simulink model "rst_auto_reg_complete_4a_2018b"  (R2018b)
settings: Solver=FixedStepAuto  StartTime=0.0  StopTime=200  RelTol=1e-3
values from neighbouring files (symbols this model uses):
  A = dend    [RST_2ordem_final.m]    (also in RST_4ordem_final.m)
  B = numd    [RST_2ordem_final.m]    (also in RST_4ordem_final.m)
  ep = 0.7    [RST_2ordem_final.m]    (also in RST_4ordem_final.m)
  initial_theta = [-0.31 -0.55 0.0021 0.12]    [RST_2ordem_final.m]    (also in RST_4ordem_final.m = [-1.0 0.38 0.07 0.23 0.03 0.12 0.06 0.005])
  Ta = 0.1    [RST_2ordem_final.m]    (also in RST_4ordem_final.m = 1)
  Tas = Ta    (= 0.1)    [RST_2ordem_final.m]    (also in RST_4ordem_final.m = 1)
  theta_switch_time = 10*Ta    (= 1)    [RST_2ordem_final.m]    (also in RST_4ordem_final.m = 10)
  Ts = 1    [RST_2ordem_final.m]    (also in RST_4ordem_final.m = 5)
  w0 = 1    [RST_2ordem_final.m]    (also in RST_4ordem_final.m = 0.1)
undefined symbols (not defined in the file or in its folder): R, S, T
libraries: dspinverses x6, simulink x2
(part 1 of 2)
settings Model: Creator=tarci  LastModifiedBy=root
settings DebuggingCC: LibraryContextMissingDiagnostic=none
settings SFSimCC: SimUseLocalCustomCode=off
settings RTWCC: RTWUseLocalCustomCode=off

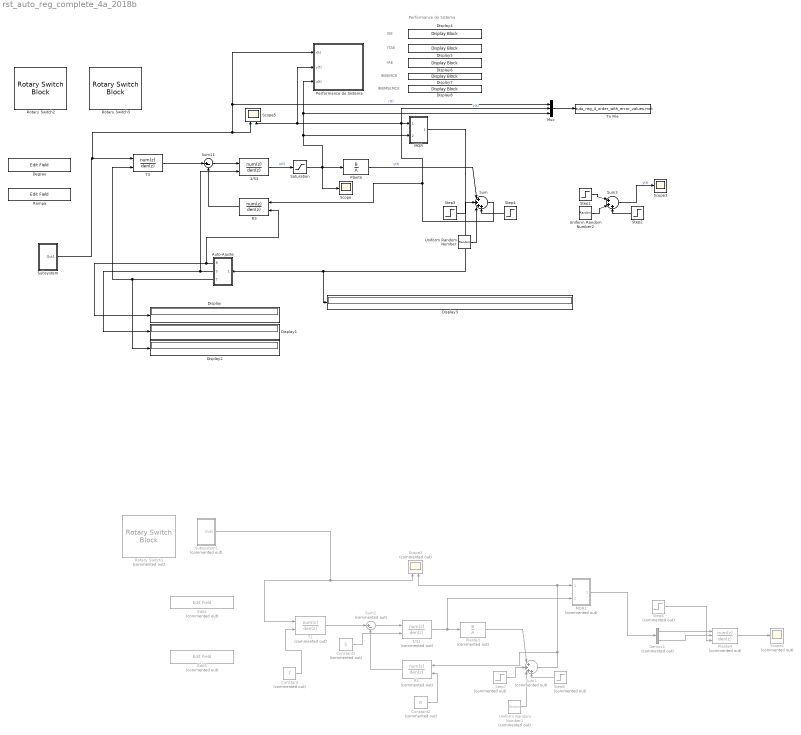
== system rst_auto_reg_complete_4a_2018b ==
  note: IRBEMCE
  note: IAE
  note: ITAE
  note: ISE
  note: Performance do Sistema
  note: IRBMSEMCE
  1/S1 : DiscreteFilter  Commented=on  Numerator=1  DenominatorSource=Input port  Denominator=1  SampleTime=Ta  a0EqualsOne=on
      settings: InputPortMap=u0,p3
  1/S3 : DiscreteFilter  Numerator=1  DenominatorSource=Input port  Denominator=1  SampleTime=Ta  a0EqualsOne=on
      settings: InputPortMap=u0,p3
  Auto-Ajuste : Subsystem
  Constant : Constant  Commented=on  Value=T
  Constant1 : Constant  Commented=on  Value=S
  Constant2 : Constant  Commented=on  Value=R
  Degrau : EditField  WebBlockId=1084  LabelPosition=Hide  Alignment=Center
  Demux1 : Demux  Commented=on  Outputs=2
  Display{,1..3} (4 alike) : Display
  Display4 : DisplayBlock  WebBlockId=2030  LabelPosition=Hide
  Display5 : DisplayBlock  WebBlockId=2031  LabelPosition=Hide
  Display6 : DisplayBlock  WebBlockId=2032  LabelPosition=Hide
  Display7 : DisplayBlock  WebBlockId=2033  LabelPosition=Hide
  Display8 : DisplayBlock  WebBlockId=2034  LabelPosition=Hide
  Edit2 : EditField  Commented=on  WebBlockId=1838  LabelPosition=Hide  Alignment=Center
  Edit3 : EditField  Commented=on  WebBlockId=1839  LabelPosition=Hide  Alignment=Center
  MQR : Subsystem
  MQR1 : Subsystem  Commented=on
  Mux : Mux  Inputs=3
  Performance do Sistema : Subsystem
  Planta : DiscreteFilter  Numerator=B  Denominator=A  SampleTime=Ta  a0EqualsOne=on
  Planta3 : DiscreteFilter  Commented=on  Numerator=B  Denominator=A  SampleTime=Ta  a0EqualsOne=on
  Planta4 : DiscreteFilter  Commented=on  NumeratorSource=Input port  Numerator=B  DenominatorSource=Input port  Denominator=A  SampleTime=Ta  a0EqualsOne=on
      settings: InputPortMap=u0,p1,p3
  R1 : DiscreteFilter  Commented=on  NumeratorSource=Input port  Numerator=[-620.2 131.3]  Denominator=1  SampleTime=Ta
      settings: InputPortMap=u0,p1
  R3 : DiscreteFilter  NumeratorSource=Input port  Numerator=[-620.2 131.3]  Denominator=1  SampleTime=Ta
      settings: InputPortMap=u0,p1
  Rampa : EditField  WebBlockId=1415  LabelPosition=Hide  Alignment=Center
  Rotary Switch1 : RotarySwitchBlock  Commented=on  WebBlockId=1942
      settings: Values={{'Degrau', 'Rampa', 'Senoide'}, [1 2 3]}
  Rotary Switch2 : RotarySwitchBlock  WebBlockId=1006
      settings: Values={{'Degrau', 'Rampa', 'Senoide'}, [1 2 3]}
  Rotary Switch3 : RotarySwitchBlock  WebBlockId=1934
      settings: Values={{'Degrau', 'Rampa', 'Senoide'}, [1 2 3]}
  Saturation : Saturate  UpperLimit=41  LowerLimit=0
  Scope : Scope
  Scope1 : Scope  Commented=on
  Scope2 : Scope  Commented=on  NumInputPorts=2
  Scope3 : Scope
  Scope5 : Scope  NumInputPorts=2
  Step1 : Step  Time=150  SampleTime=0
  Step2 : Step  Time=151  After=-1  SampleTime=0
  Step3 : Step  Time=150  SampleTime=0
  Step4 : Step  Time=151  After=-1  SampleTime=0
  Step6 : Step  Commented=on  SampleTime=0
  Step7 : Step  Commented=on  Time=40  SampleTime=0
  Step8 : Step  Commented=on  Time=41  After=-1  SampleTime=0
  Subsystem : Subsystem
  Subsystem1 : Subsystem  Commented=on
  Sum : Sum  Inputs=|++++
  Sum1 : Sum  Commented=on  Inputs=|++++
  Sum11 : Sum  Inputs=|+-
  Sum2 : Sum  Commented=on  Inputs=|+-
  Sum3 : Sum  Inputs=|+++
  T1 : DiscreteFilter  Commented=on  NumeratorSource=Input port  Numerator=13.39  Denominator=1  SampleTime=Ta
      settings: InputPortMap=u0,p1
  T3 : DiscreteFilter  NumeratorSource=Input port  Numerator=13.39  Denominator=1  SampleTime=Ta
      settings: InputPortMap=u0,p1
  To File : ToFile  Filename=auto_reg_4_order_with_error_values.mat
  Uniform Random Number : UniformRandomNumber  Minimum=-0.1  Maximum=0.1  Seed=10  SampleTime=0
  Uniform Random Number1 : UniformRandomNumber  Commented=on  Minimum=-0.1  Maximum=0.1  SampleTime=0
  Uniform Random Number2 : UniformRandomNumber  Minimum=-0.1  Maximum=0.1  Seed=10  SampleTime=0
  wires:
  Sum11/1 -> 1/S3/1
  R3/1 -> Sum11/2
  T3/1 -> Sum11/1
  Auto-Ajuste/1(R) -> Display/1, R3/2
  Auto-Ajuste/2(S) -> Display1/1, 1/S3/2
  Auto-Ajuste/3(T) -> Display2/1, T3/2
  MQR/1("Theta(t) ") -> Display3/1, Auto-Ajuste/1(Theta)
  Step3/1 -> Sum/2
  Step4/1 -> Sum/4
  Uniform Random Number/1 -> Sum/3
  Step8/1 -> Sum1/4
  Step7/1 -> Sum1/2
  1/S1/1 -> MQR1/2("u(t) "), Planta3/1
  Uniform Random Number1/1 -> Sum1/3
  Step6/1 -> Planta4/1
  Planta4/1 -> Scope1/1
  Demux1/2 -> Planta4/2
  Sum1/1 -> R1/1, Scope2/2, MQR1/1(y(t))
  R1/1 -> Sum2/2
  Subsystem1/1(Out1) -> T1/1, Scope2/1
  T1/1 -> Sum2/1
  Demux1/1 -> Planta4/3
  Sum2/1 -> 1/S1/1
  MQR1/1("Theta(t) ") -> Demux1/1
  Planta3/1 -> Sum1/1
  Constant/1 -> T1/2
  Constant1/1 -> 1/S1/2
  Constant2/1 -> R1/2
  Subsystem/1(Out1) -> Performance do Sistema/1(r(t)), Mux/1, Scope5/1, T3/1  "r(t)"
  1/S3/1 -> Saturation/1  "u(t)"
  Mux/1 -> To File/1
  Saturation/1 -> MQR/2("u(t) "), Mux/3, Performance do Sistema/3(u(t)), Planta/1, Scope/1
  Planta/1 -> Sum/1  "y(t)"
  Sum/1 -> R3/1, Scope5/2, Performance do Sistema/2(y(t)), Mux/2, MQR/1(y(t))  "y(t)"
  Step1/1 -> Sum3/1
  Uniform Random Number2/1 -> Sum3/2
  Step2/1 -> Sum3/3
  Sum3/1 -> Scope3/1  "y(t)"

== system rst_auto_reg_complete_4a_2018b/Auto-Ajuste ==
  Theta : Inport
  Damping3 : Constant  Value=ep
  Display : Display
  Display1 : Display
  Display2 : Display
  Frequência : Constant  Value=w0
  MC : Constant
  Multiport Switch : MultiPortSwitch
  Multiport Switch1 : MultiPortSwitch
  Multiport Switch2 : MultiPortSwitch
  RST Degrau : Subsystem
  RST Rampa : Subsystem
  RST Senoide : Subsystem
  Sample Time 2 : Constant  Value=Tas
  Sample Time3 : Constant  Value=Ta
  Ts3 : Constant  Value=Ts
  R : Outport
  S : Outport  Port=2
  T : Outport  Port=3
  wires:
  RST Senoide/4(L) -> Display2/1
  RST Degrau/4(L) -> Display1/1
  RST Rampa/2(S) -> Multiport Switch1/3
  RST Senoide/3(T) -> Multiport Switch2/4
  RST Rampa/4(L) -> Display/1
  Multiport Switch2/1 -> T/1
  Multiport Switch1/1 -> S/1
  Multiport Switch/1 -> R/1
  RST Senoide/1(R) -> Multiport Switch/4
  Ts3/1 -> RST Degrau/2(Ts), RST Rampa/2(Ts), RST Senoide/2(Ts)
  RST Degrau/2(S) -> Multiport Switch1/2
  RST Senoide/2(S) -> Multiport Switch1/4
  RST Rampa/1(R) -> Multiport Switch/3
  Frequência/1 -> RST Senoide/5(w0)
  Sample Time 2/1 -> RST Senoide/6(Tas)
  Sample Time3/1 -> RST Degrau/1(Sample Time), RST Rampa/1(Sample Time), RST Senoide/1(Sample Time)
  RST Rampa/3(T) -> Multiport Switch2/3
  Theta/1 -> RST Degrau/4(Theta), RST Rampa/4(Theta), RST Senoide/4(Theta)
  RST Degrau/3(T) -> Multiport Switch2/2
  Damping3/1 -> RST Degrau/3(Damping), RST Rampa/3(Damping), RST Senoide/3(Damping)
  RST Degrau/1(R) -> Multiport Switch/2
  MC/1 -> Multiport Switch/1, Multiport Switch1/1, Multiport Switch2/1

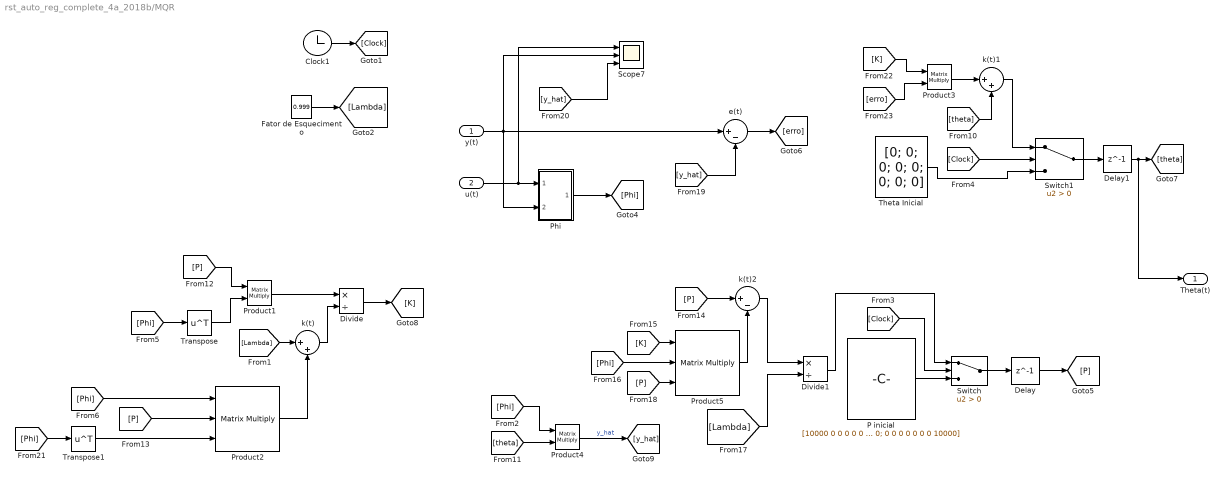
== system rst_auto_reg_complete_4a_2018b/MQR ==
  y(t) : Inport
  "u(t) " : Inport  Port=2
  Clock1 : Clock
  Delay : Delay  DelayLength=1  InitialCondition=0
  Delay1 : Delay  DelayLength=1  InitialCondition=0
  Divide : Product  Inputs=*/
  Divide1 : Product  Inputs=*/
  "Fator de Esquecimento " : Constant  Value=0.999
  P inicial : Constant  Value=[10000 0 0 0 0 0 0 0; 0 10000 0 0 0 0 0 0; 0 0 10000 0 0 0 0 0; 0 0 0 10000 0 0 0 0; 0 0 0 0 10000 0 0 0; 0 0 0 0 0 10000 0 0; 0 0 0 0 0 0 10000 0; 0 0 0 0 0 0 0 10000]
  Phi : Subsystem
  Product1 : Product  Multiplication=Matrix(*)
  Product2 : Product  Inputs=3  Multiplication=Matrix(*)
  Product3 : Product  Multiplication=Matrix(*)
  Product4 : Product  Multiplication=Matrix(*)
  Product5 : Product  Inputs=3  Multiplication=Matrix(*)
  Scope7 : Scope  NumInputPorts=3
  Switch : Switch  Criteria=u2 > Threshold
  Switch1 : Switch  Criteria=u2 > Threshold
  "Theta Inicial " : Constant  Value=[0; 0; 0; 0; 0; 0; 0; 0]
  Transpose : Math  Operator=transpose  SaturateOnIntegerOverflow=on
  Transpose1 : Math  Operator=transpose  SaturateOnIntegerOverflow=on
  e(t) : Sum  Inputs=|+-
  k(t) : Sum  Inputs=|++
  k(t)1 : Sum  Inputs=|++
  k(t)2 : Sum  Inputs=|+-
  "Theta(t) " : Outport
  wires:
  Product4/1 -> [y_hat]  "y_hat"
  [Phi] -> Product5/2
  Divide/1 -> [K]
  [Phi] -> Product2/1
  [P] -> Product1/1
  P inicial/1 -> Switch/3
  [K] -> Product5/1
  [y_hat] -> e(t)/2
  [erro] -> Product3/2
  Clock1/1 -> [Clock]
  Transpose/1 -> Product1/2
  [Lambda] -> k(t)/1
  [P] -> Product2/2
  [theta] -> k(t)1/2
  [P] -> k(t)2/1
  [theta] -> Product4/2
  [Clock] -> Switch/2
  [Phi] -> Transpose/1
  Divide1/1 -> Switch/1
  Transpose1/1 -> Product2/3
  "Theta Inicial "/1 -> Switch1/3
  "Fator de Esquecimento "/1 -> [Lambda]
  [P] -> Product5/3
  [Phi] -> Transpose1/1
  Delay/1 -> [P]
  Product3/1 -> k(t)1/1
  e(t)/1 -> [erro]
  Product1/1 -> Divide/1
  [Lambda] -> Divide1/2
  Switch/1 -> Delay/1
  "u(t) "/1 -> Phi/1(u(t)), Scope7/1
  Product5/1 -> k(t)2/2
  Delay1/1 -> [theta], "Theta(t) "/1
  k(t)2/1 -> Divide1/1
  y(t)/1 -> Phi/2(y(t)), Scope7/2, e(t)/1
  [Clock] -> Switch1/2
  Product2/1 -> k(t)/2
  [K] -> Product3/1
  Switch1/1 -> Delay1/1
  [y_hat] -> Scope7/3
  k(t)1/1 -> Switch1/1
  Phi/1(Phi) -> [Phi]
  [Phi] -> Product4/1
  k(t)/1 -> Divide/2

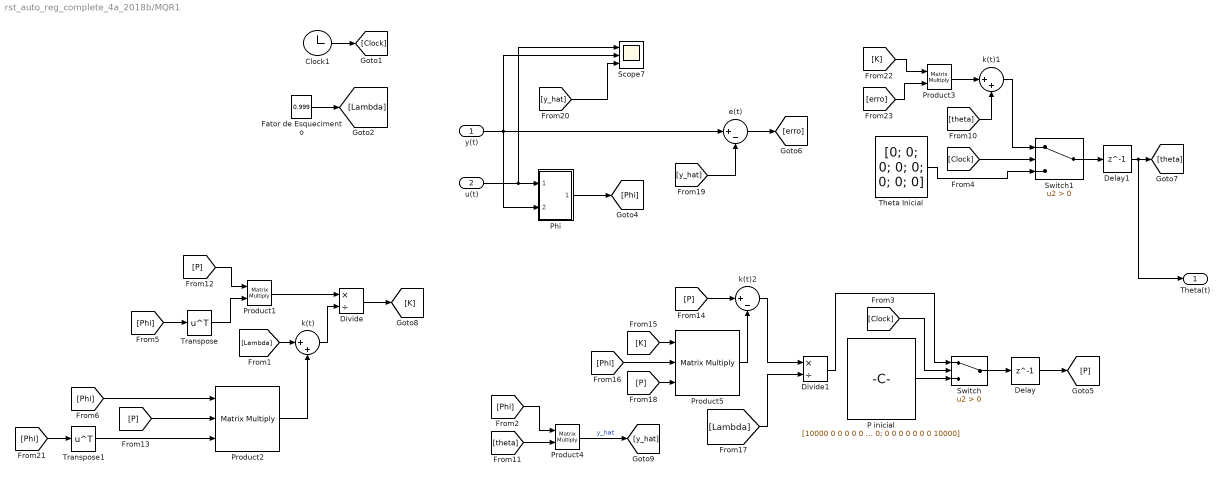
== system rst_auto_reg_complete_4a_2018b/MQR1 ==
  y(t) : Inport
  "u(t) " : Inport  Port=2
  Clock1 : Clock
  Delay : Delay  DelayLength=1  InitialCondition=0
  Delay1 : Delay  DelayLength=1  InitialCondition=0
  Divide : Product  Inputs=*/
  Divide1 : Product  Inputs=*/
  "Fator de Esquecimento " : Constant  Value=0.999
  P inicial : Constant  Value=[10000 0 0 0 0 0 0 0; 0 10000 0 0 0 0 0 0; 0 0 10000 0 0 0 0 0; 0 0 0 10000 0 0 0 0; 0 0 0 0 10000 0 0 0; 0 0 0 0 0 10000 0 0; 0 0 0 0 0 0 10000 0; 0 0 0 0 0 0 0 10000]
  Phi : Subsystem
  Product1 : Product  Multiplication=Matrix(*)
  Product2 : Product  Inputs=3  Multiplication=Matrix(*)
  Product3 : Product  Multiplication=Matrix(*)
  Product4 : Product  Multiplication=Matrix(*)
  Product5 : Product  Inputs=3  Multiplication=Matrix(*)
  Scope7 : Scope  NumInputPorts=3
  Switch : Switch  Criteria=u2 > Threshold
  Switch1 : Switch  Criteria=u2 > Threshold
  "Theta Inicial " : Constant  Value=[0; 0; 0; 0; 0; 0; 0; 0]
  Transpose : Math  Operator=transpose  SaturateOnIntegerOverflow=on
  Transpose1 : Math  Operator=transpose  SaturateOnIntegerOverflow=on
  e(t) : Sum  Inputs=|+-
  k(t) : Sum  Inputs=|++
  k(t)1 : Sum  Inputs=|++
  k(t)2 : Sum  Inputs=|+-
  "Theta(t) " : Outport
  wires:
  Product4/1 -> [y_hat]  "y_hat"
  [Phi] -> Product5/2
  Divide/1 -> [K]
  [Phi] -> Product2/1
  [P] -> Product1/1
  P inicial/1 -> Switch/3
  [K] -> Product5/1
  [y_hat] -> e(t)/2
  [erro] -> Product3/2
  Clock1/1 -> [Clock]
  Transpose/1 -> Product1/2
  [Lambda] -> k(t)/1
  [P] -> Product2/2
  [theta] -> k(t)1/2
  [P] -> k(t)2/1
  [theta] -> Product4/2
  [Clock] -> Switch/2
  [Phi] -> Transpose/1
  Divide1/1 -> Switch/1
  Transpose1/1 -> Product2/3
  "Theta Inicial "/1 -> Switch1/3
  "Fator de Esquecimento "/1 -> [Lambda]
  [P] -> Product5/3
  [Phi] -> Transpose1/1
  Delay/1 -> [P]
  Product3/1 -> k(t)1/1
  e(t)/1 -> [erro]
  Product1/1 -> Divide/1
  [Lambda] -> Divide1/2
  Switch/1 -> Delay/1
  "u(t) "/1 -> Phi/1(u(t)), Scope7/1
  Product5/1 -> k(t)2/2
  Delay1/1 -> [theta], "Theta(t) "/1
  k(t)2/1 -> Divide1/1
  y(t)/1 -> Phi/2(y(t)), Scope7/2, e(t)/1
  [Clock] -> Switch1/2
  Product2/1 -> k(t)/2
  [K] -> Product3/1
  Switch1/1 -> Delay1/1
  [y_hat] -> Scope7/3
  k(t)1/1 -> Switch1/1
  Phi/1(Phi) -> [Phi]
  [Phi] -> Product4/1
  k(t)/1 -> Divide/2

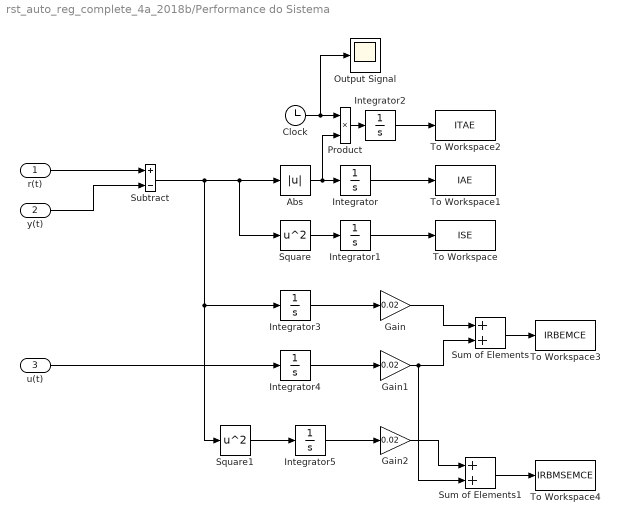
== system rst_auto_reg_complete_4a_2018b/Performance do Sistema ==
  r(t) : Inport
  y(t) : Inport  Port=2
  u(t) : Inport  Port=3
  Abs : Abs
  Clock : Clock
  Gain : Gain  Gain=0.02
  Gain1 : Gain  Gain=0.02
  Gain2 : Gain  Gain=0.02
  Integrator{,1..5} (6 alike) : Integrator
  Output Signal : Scope
  Product : Product
  Square : Math  Operator=square  SaturateOnIntegerOverflow=on
  Square1 : Math  Operator=square  SaturateOnIntegerOverflow=on
  Subtract : Sum  Inputs=+-
  Sum of Elements : Sum
  Sum of Elements1 : Sum
  To Workspace : ToWorkspace  VariableName=ISE  SaveFormat=Timeseries  SampleTime=-1
  To Workspace1 : ToWorkspace  VariableName=IAE  SaveFormat=Timeseries  SampleTime=-1
  To Workspace2 : ToWorkspace  VariableName=ITAE  SaveFormat=Timeseries  SampleTime=-1
  To Workspace3 : ToWorkspace  VariableName=IRBEMCE  SaveFormat=Timeseries  SampleTime=-1
  To Workspace4 : ToWorkspace  VariableName=IRBMSEMCE  SaveFormat=Timeseries  SampleTime=-1
  wires:
  y(t)/1 -> Subtract/2
  Abs/1 -> Product/2, Integrator/1
  Integrator/1 -> To Workspace1/1
  Integrator1/1 -> To Workspace/1
  Square/1 -> Integrator1/1
  Clock/1 -> Output Signal/1, Product/1
  Product/1 -> Integrator2/1
  Integrator2/1 -> To Workspace2/1
  r(t)/1 -> Subtract/1
  Subtract/1 -> Square1/1, Integrator3/1, Square/1, Abs/1
  Integrator3/1 -> Gain/1
  Integrator4/1 -> Gain1/1
  Gain/1 -> Sum of Elements/1
  Gain1/1 -> Sum of Elements1/2, Sum of Elements/2
  Square1/1 -> Integrator5/1
  Integrator5/1 -> Gain2/1
  Gain2/1 -> Sum of Elements1/1
  Sum of Elements/1 -> To Workspace3/1
  Sum of Elements1/1 -> To Workspace4/1
  u(t)/1 -> Integrator4/1

== system rst_auto_reg_complete_4a_2018b/Subsystem ==
  Constant3 : Constant
  Multiport Switch : MultiPortSwitch
  Ramp : simulink/Sources/Ramp  slope=1  start=1  InitialOutput=0
  Sine Wave : Sin  Frequency=w0  SampleTime=Tas
  Step1 : Step  Time=0  SampleTime=0
  Step2 : Step  Time=30  After=2  SampleTime=0
  Step3 : Step  Time=60  After=-3  SampleTime=0
  Step4 : Step  Time=90  After=4  SampleTime=0
  Step5 : Step  Time=120  After=-2  SampleTime=0
  Sum : Sum  Inputs=|+++++
  Out1 : Outport
  wires:
  Sine Wave/1 -> Multiport Switch/4
  Sum/1 -> Multiport Switch/2
  Constant3/1 -> Multiport Switch/1
  Ramp/1 -> Multiport Switch/3
  Multiport Switch/1 -> Out1/1
  Step2/1 -> Sum/2
  Step3/1 -> Sum/3
  Step1/1 -> Sum/1
  Step5/1 -> Sum/5
  Step4/1 -> Sum/4

== system rst_auto_reg_complete_4a_2018b/Subsystem1 ==
  C2 : Constant  Value=2
  Multiport Switch : MultiPortSwitch
  Ramp : simulink/Sources/Ramp  slope=1  start=1  InitialOutput=0
  Sine Wave : Sin  Frequency=w0  SampleTime=Tas
  Step1 : Step  Time=0  SampleTime=0
  Out1 : Outport
  wires:
  Multiport Switch/1 -> Out1/1
  Ramp/1 -> Multiport Switch/3
  C2/1 -> Multiport Switch/1
  Step1/1 -> Multiport Switch/2
  Sine Wave/1 -> Multiport Switch/4

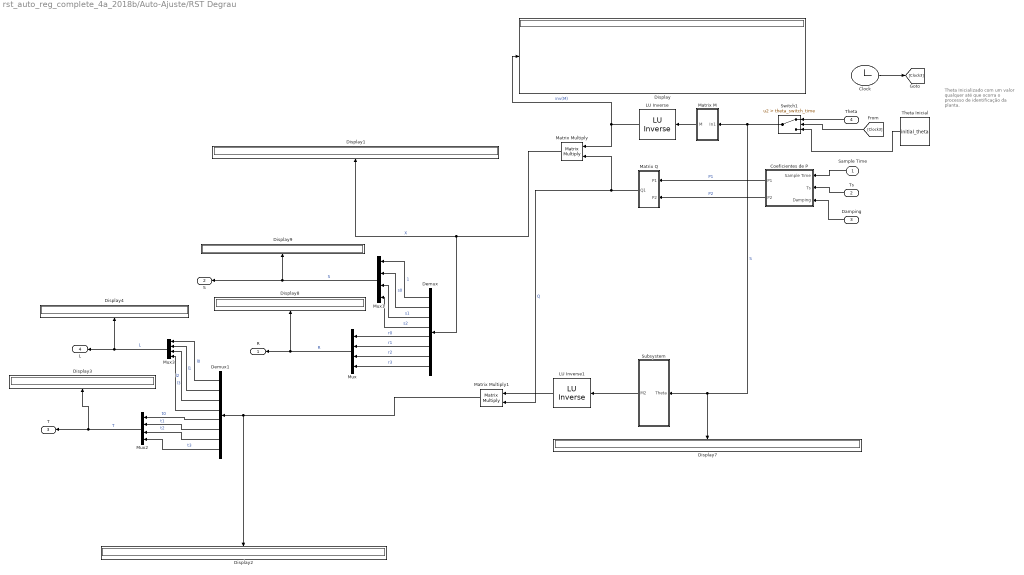
== system rst_auto_reg_complete_4a_2018b/Auto-Ajuste/RST Degrau ==
  note: Theta Inicializado com um
      | valor qualquer até que ocorra
      |  o processo de identificação
      | da planta.
  Sample Time : Inport
  Ts : Inport  Port=2
  Damping : Inport  Port=3
  Theta : Inport  Port=4
  " LU Inverse" : dspinverses/ LU Inverse
      settings: SourceProductName=DSP System Toolbox
  " LU Inverse1" : dspinverses/ LU Inverse
      settings: SourceProductName=DSP System Toolbox
  Clock : Clock
  Coeficientes de P : Subsystem
  Demux : Demux  Outputs=8
  Demux1 : Demux  Outputs=8
  Display{,1..4,7..9} (8 alike) : Display
  Matrix M : Subsystem
  Matrix Multiply : Product  Multiplication=Matrix(*)
  Matrix Multiply1 : Product  Multiplication=Matrix(*)
  Matrix Q : Subsystem
  Mux{,1..3} (4 alike) : Mux
  Subsystem : Subsystem
  Switch1 : Switch  Criteria=u2 > Threshold  Threshold=theta_switch_time
  Theta Inicial : Constant  Value=initial_theta
  R : Outport
  S : Outport  Port=2
  T : Outport  Port=3
  L : Outport  Port=4
  wires:
  Matrix Multiply1/1 -> Demux1/1, Display2/1
  Demux1/1 -> Mux3/1  "l0"
  Mux3/1 -> Display4/1, L/1  "L"
  Demux1/2 -> Mux3/2  "l1"
  Mux2/1 -> Display3/1, T/1  "T"
  Subsystem/1(M2) -> " LU Inverse1"/1
  Matrix Q/1(Q1) -> Matrix Multiply/2, Matrix Multiply1/2  "Q"
  " LU Inverse1"/1 -> Matrix Multiply1/1
  Demux/2 -> Mux1/2  "s0"
  Demux/1 -> Mux1/1  "1"
  Matrix M/1(M) -> " LU Inverse"/1
  Theta Inicial/1 -> Switch1/3
  [Clock3] -> Switch1/2
  Theta/1 -> Switch1/1
  Switch1/1 -> Subsystem/1(Theta), Display7/1, Matrix M/1(In1)  "S"
  Clock/1 -> [Clock3]
  Mux/1 -> Display8/1, R/1  "R"
  Coeficientes de P/1(P1) -> Matrix Q/1(P1)  "P1"
  Sample Time/1 -> Coeficientes de P/1(Sample Time)
  Damping/1 -> Coeficientes de P/3(Damping)
  Ts/1 -> Coeficientes de P/2(Ts)
  Coeficientes de P/2(P2) -> Matrix Q/2(P2)  "P2"
  Mux1/1 -> S/1, Display9/1  "S"
  " LU Inverse"/1 -> Display/1, Matrix Multiply/1  "inv(M)"
  Matrix Multiply/1 -> Display1/1, Demux/1  "X"
  Demux/3 -> Mux1/3  "s1"
  Demux/4 -> Mux1/4  "s2"
  Demux/5 -> Mux/1  "r0"
  Demux/6 -> Mux/2  "r1"
  Demux/7 -> Mux/3  "r2"
  Demux/8 -> Mux/4  "r3"
  Demux1/3 -> Mux3/3  "l2"
  Demux1/4 -> Mux3/4  "l3"
  Demux1/5 -> Mux2/1  "t0"
  Demux1/6 -> Mux2/2  "t1"
  Demux1/7 -> Mux2/3  "t2"
  Demux1/8 -> Mux2/4  "t3"

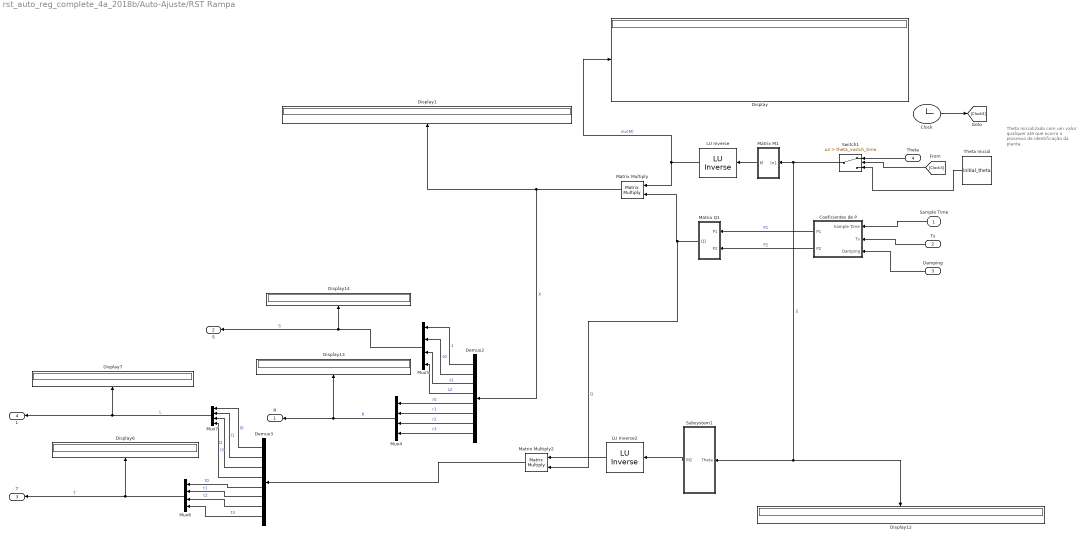
== system rst_auto_reg_complete_4a_2018b/Auto-Ajuste/RST Rampa ==
  note: Theta Inicializado com um
      | valor qualquer até que ocorra
      |  o processo de identificação
      | da planta.
  Sample Time : Inport
  Ts : Inport  Port=2
  Damping : Inport  Port=3
  Theta : Inport  Port=4
  " LU Inverse" : dspinverses/ LU Inverse
      settings: SourceProductName=DSP System Toolbox
  " LU Inverse2" : dspinverses/ LU Inverse
      settings: SourceProductName=DSP System Toolbox
  Clock : Clock
  Coeficientes de P : Subsystem
  Demux2 : Demux  Outputs=8
  Demux3 : Demux  Outputs=8
  Display{,1,6..7,12..14} (7 alike) : Display
  Matrix M1 : Subsystem
  Matrix Multiply : Product  Multiplication=Matrix(*)
  Matrix Multiply2 : Product  Multiplication=Matrix(*)
  Matrix Q1 : Subsystem
  Mux{4..7} (4 alike) : Mux
  Subsystem1 : Subsystem
  Switch1 : Switch  Criteria=u2 > Threshold  Threshold=theta_switch_time
  Theta Inicial : Constant  Value=initial_theta
  R : Outport
  S : Outport  Port=2
  T : Outport  Port=3
  L : Outport  Port=4
  wires:
  " LU Inverse"/1 -> Matrix Multiply/1, Display/1  "inv(M)"
  Coeficientes de P/2(P2) -> Matrix Q1/2(P2)  "P2"
  Ts/1 -> Coeficientes de P/2(Ts)
  Damping/1 -> Coeficientes de P/3(Damping)
  Sample Time/1 -> Coeficientes de P/1(Sample Time)
  Coeficientes de P/1(P1) -> Matrix Q1/1(P1)  "P1"
  Clock/1 -> [Clock3]
  Theta/1 -> Switch1/1
  [Clock3] -> Switch1/2
  Theta Inicial/1 -> Switch1/3
  Matrix M1/1(M) -> " LU Inverse"/1
  Demux3/3 -> Mux7/3  "l2"
  Demux2/8 -> Mux4/4  "r3"
  Demux2/5 -> Mux4/1  "r0"
  Demux2/4 -> Mux5/4  "s2"
  Demux3/2 -> Mux7/2  "l1"
  Demux2/3 -> Mux5/3  "s1"
  Demux3/8 -> Mux6/4  "t3"
  Demux3/5 -> Mux6/1  "t0"
  Mux4/1 -> Display13/1, R/1  "R"
  Switch1/1 -> Subsystem1/1(Theta), Display12/1, Matrix M1/1(In1)  "S"
  Demux2/2 -> Mux5/2  "s0"
  Mux5/1 -> Display14/1, S/1  "S"
  " LU Inverse2"/1 -> Matrix Multiply2/1
  Matrix Multiply/1 -> Demux2/1, Display1/1  "X"
  Demux3/7 -> Mux6/3  "t2"
  Demux2/1 -> Mux5/1  "1"
  Mux7/1 -> Display7/1, L/1  "L"
  Matrix Multiply2/1 -> Demux3/1
  Demux3/1 -> Mux7/1  "l0"
  Subsystem1/1(M2) -> " LU Inverse2"/1
  Matrix Q1/1(Q1) -> Matrix Multiply2/2, Matrix Multiply/2  "Q"
  Demux3/6 -> Mux6/2  "t1"
  Demux2/7 -> Mux4/3  "r2"
  Demux3/4 -> Mux7/4  "l3"
  Mux6/1 -> Display6/1, T/1  "T"
  Demux2/6 -> Mux4/2  "r1"

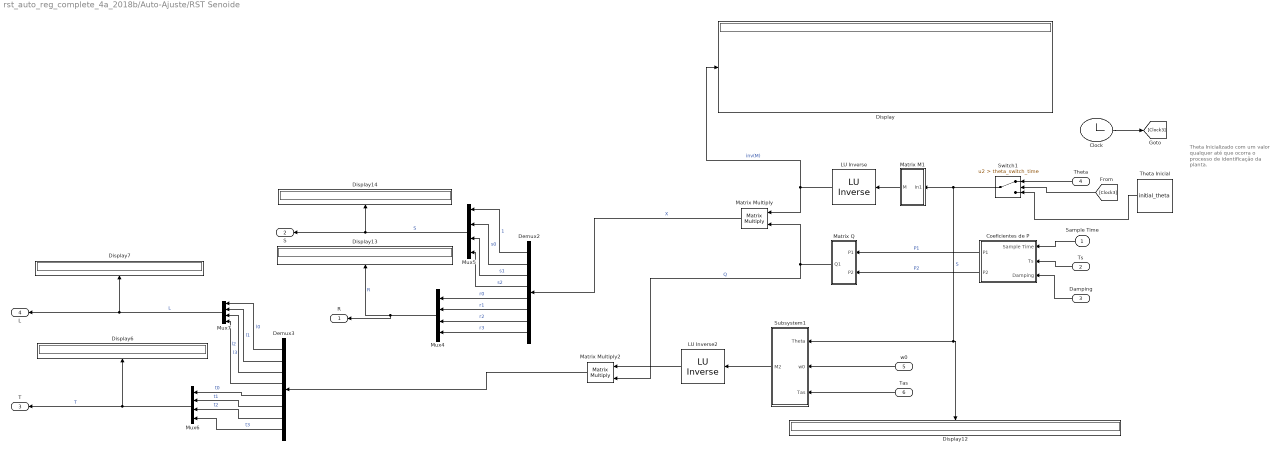
== system rst_auto_reg_complete_4a_2018b/Auto-Ajuste/RST Senoide ==
  note: Theta Inicializado com um
      | valor qualquer até que ocorra
      |  o processo de identificação
      | da planta.
  Sample Time : Inport
  Ts : Inport  Port=2
  Damping : Inport  Port=3
  Theta : Inport  Port=4
  w0 : Inport  Port=5
  Tas : Inport  Port=6
  " LU Inverse" : dspinverses/ LU Inverse
      settings: SourceProductName=DSP System Toolbox
  " LU Inverse2" : dspinverses/ LU Inverse
      settings: SourceProductName=DSP System Toolbox
  Clock : Clock
  Coeficientes de P : Subsystem
  Demux2 : Demux  Outputs=8
  Demux3 : Demux  Outputs=8
  Display{,6..7,12..14} (6 alike) : Display
  Matrix M1 : Subsystem
  Matrix Multiply : Product  Multiplication=Matrix(*)
  Matrix Multiply2 : Product  Multiplication=Matrix(*)
  Matrix Q : Subsystem
  Mux{4..7} (4 alike) : Mux
  Subsystem1 : Subsystem
  Switch1 : Switch  Criteria=u2 > Threshold  Threshold=theta_switch_time
  Theta Inicial : Constant  Value=initial_theta
  R : Outport
  S : Outport  Port=2
  T : Outport  Port=3
  L : Outport  Port=4
  wires:
  Tas/1 -> Subsystem1/3(Tas)
  w0/1 -> Subsystem1/2(w0)
  " LU Inverse"/1 -> Matrix Multiply/1, Display/1  "inv(M)"
  Coeficientes de P/2(P2) -> Matrix Q/2(P2)  "P2"
  Ts/1 -> Coeficientes de P/2(Ts)
  Damping/1 -> Coeficientes de P/3(Damping)
  Sample Time/1 -> Coeficientes de P/1(Sample Time)
  Coeficientes de P/1(P1) -> Matrix Q/1(P1)  "P1"
  Clock/1 -> [Clock3]
  Theta/1 -> Switch1/1
  [Clock3] -> Switch1/2
  Theta Inicial/1 -> Switch1/3
  Matrix M1/1(M) -> " LU Inverse"/1
  Demux3/3 -> Mux7/3  "l2"
  Demux2/8 -> Mux4/4  "r3"
  Demux2/5 -> Mux4/1  "r0"
  Demux2/4 -> Mux5/4  "s2"
  Demux3/2 -> Mux7/2  "l1"
  Demux2/3 -> Mux5/3  "s1"
  Demux3/8 -> Mux6/4  "t3"
  Demux3/5 -> Mux6/1  "t0"
  Mux4/1 -> Display13/1, R/1  "R"
  Switch1/1 -> Subsystem1/1(Theta), Display12/1, Matrix M1/1(In1)  "S"
  Demux2/2 -> Mux5/2  "s0"
  Mux5/1 -> Display14/1, S/1  "S"
  " LU Inverse2"/1 -> Matrix Multiply2/1
  Matrix Multiply/1 -> Demux2/1  "X"
  Demux3/7 -> Mux6/3  "t2"
  Demux2/1 -> Mux5/1  "1"
  Mux7/1 -> Display7/1, L/1  "L"
  Matrix Multiply2/1 -> Demux3/1
  Demux3/1 -> Mux7/1  "l0"
  Subsystem1/1(M2) -> " LU Inverse2"/1
  Matrix Q/1(Q1) -> Matrix Multiply/2, Matrix Multiply2/2  "Q"
  Demux3/6 -> Mux6/2  "t1"
  Demux2/7 -> Mux4/3  "r2"
  Demux3/4 -> Mux7/4  "l3"
  Mux6/1 -> Display6/1, T/1  "T"
  Demux2/6 -> Mux4/2  "r1"

== system rst_auto_reg_complete_4a_2018b/MQR/Phi ==
  u(t) : Inport
  y(t) : Inport  Port=2
  Constant : Constant  Value=-1
  Delay : Delay
  Delay1 : Delay  DelayLength=1
  Delay2 : Delay
  Delay3 : Delay  DelayLength=1
  Delay4 : Delay  DelayLength=3
  Delay5 : Delay  DelayLength=4
  Delay6 : Delay  DelayLength=3
  Delay7 : Delay  DelayLength=4
  Display : Display
  Product : Product
  Transpose1 : Math  Operator=transpose  SaturateOnIntegerOverflow=on
  Vector Concatenate : Concatenate  NumInputs=8
  Phi : Outport
  wires:
  Delay7/1 -> Vector Concatenate/8
  Delay6/1 -> Vector Concatenate/7
  Delay2/1 -> Vector Concatenate/6
  Delay3/1 -> Vector Concatenate/5
  Delay5/1 -> Vector Concatenate/4
  Delay4/1 -> Vector Concatenate/3
  Product/1 -> Delay1/1, Delay/1, Delay4/1, Delay5/1
  Constant/1 -> Product/2
  Transpose1/1 -> Phi/1
  Delay1/1 -> Vector Concatenate/1
  y(t)/1 -> Product/1
  Delay/1 -> Vector Concatenate/2
  Vector Concatenate/1 -> Display/1, Transpose1/1  "Phi"
  u(t)/1 -> Delay3/1, Delay2/1, Delay6/1, Delay7/1

== system rst_auto_reg_complete_4a_2018b/MQR1/Phi ==
  u(t) : Inport
  y(t) : Inport  Port=2
  Constant : Constant  Value=-1
  Delay : Delay
  Delay1 : Delay  DelayLength=1
  Delay2 : Delay
  Delay3 : Delay  DelayLength=1
  Delay4 : Delay  DelayLength=3
  Delay5 : Delay  DelayLength=4
  Delay6 : Delay  DelayLength=3
  Delay7 : Delay  DelayLength=4
  Display : Display
  Product : Product
  Transpose1 : Math  Operator=transpose  SaturateOnIntegerOverflow=on
  Vector Concatenate : Concatenate  NumInputs=8
  Phi : Outport
  wires:
  Delay7/1 -> Vector Concatenate/8
  Delay6/1 -> Vector Concatenate/7
  Delay2/1 -> Vector Concatenate/6
  Delay3/1 -> Vector Concatenate/5
  Delay5/1 -> Vector Concatenate/4
  Delay4/1 -> Vector Concatenate/3
  Product/1 -> Delay1/1, Delay/1, Delay4/1, Delay5/1
  Constant/1 -> Product/2
  Transpose1/1 -> Phi/1
  Delay1/1 -> Vector Concatenate/1
  y(t)/1 -> Product/1
  Delay/1 -> Vector Concatenate/2
  Vector Concatenate/1 -> Display/1, Transpose1/1  "Phi"
  u(t)/1 -> Delay3/1, Delay2/1, Delay6/1, Delay7/1

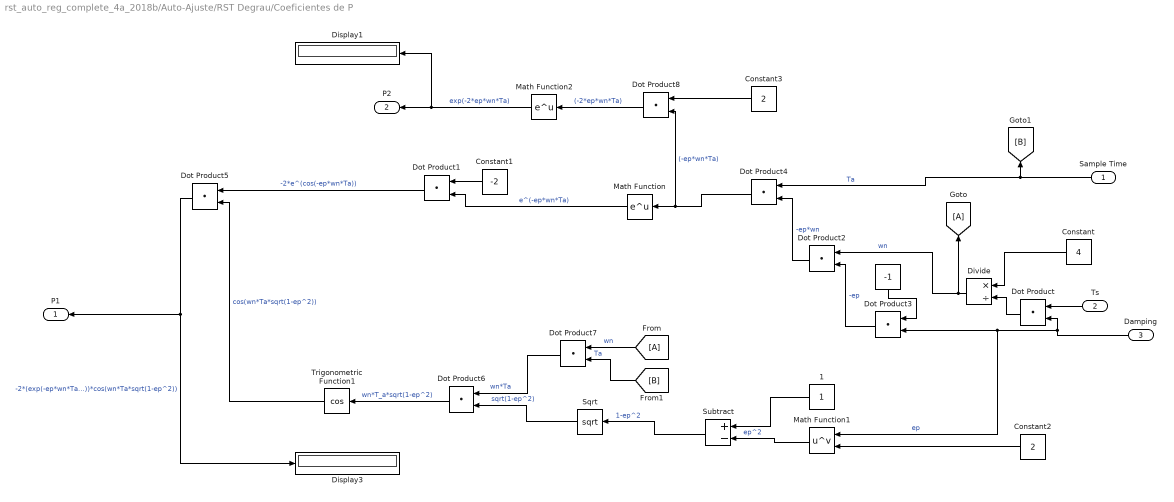
== system rst_auto_reg_complete_4a_2018b/Auto-Ajuste/RST Degrau/Coeficientes de P ==
  Sample Time : Inport
  Ts : Inport  Port=2
  Damping : Inport  Port=3
  " " : Constant  Value=-1
  1 : Constant
  Constant : Constant  Value=4
  Constant1 : Constant  Value=-2
  Constant2 : Constant  Value=2
  Constant3 : Constant  Value=2
  Display1 : Display
  Display3 : Display
  Divide : Product  Inputs=*/
  Dot Product{,1..8} (9 alike) : DotProduct  InputSameDT=on  OutDataTypeStr=Inherit: Inherit via internal rule
  Math Function : Math  SaturateOnIntegerOverflow=on
  Math Function1 : Math  Operator=pow  SaturateOnIntegerOverflow=on
  Math Function2 : Math  SaturateOnIntegerOverflow=on
  Sqrt : Sqrt  SaturateOnIntegerOverflow=on
  Subtract : Sum  Inputs=+-
  Trigonometric Function1 : Trigonometry  Operator=cos
  P1 : Outport
  P2 : Outport  Port=2
  wires:
  Math Function2/1 -> P2/1, Display1/1  "exp(-2*ep*wn*Ta)"
  Dot Product8/1 -> Math Function2/1  "(-2*ep*wn*Ta)"
  Constant3/1 -> Dot Product8/1
  Subtract/1 -> Sqrt/1  "1-ep^2"
  Sqrt/1 -> Dot Product6/2  "sqrt(1-ep^2)"
  Dot Product4/1 -> Math Function/1, Dot Product8/2  "(-ep*wn*Ta)"
  Dot Product6/1 -> Trigonometric Function1/1  "wn*T_a*sqrt(1-ep^2)"
  [B] -> Dot Product7/2  "Ta"
  Dot Product2/1 -> Dot Product4/2  "-ep*wn"
  Constant1/1 -> Dot Product1/1
  1/1 -> Subtract/1
  Constant2/1 -> Math Function1/2
  Dot Product1/1 -> Dot Product5/1  "-2*e^(cos(-ep*wn*Ta))"
  Math Function1/1 -> Subtract/2  "ep^2"
  Sample Time/1 -> [B], Dot Product4/1  "Ta"
  Dot Product7/1 -> Dot Product6/1  "wn*Ta"
  Constant/1 -> Divide/1
  Damping/1 -> Dot Product/2, Dot Product3/2, Math Function1/1  "ep"
  Dot Product3/1 -> Dot Product2/2  "-ep"
  Dot Product/1 -> Divide/2
  Ts/1 -> Dot Product/1
  Trigonometric Function1/1 -> Dot Product5/2  "cos(wn*Ta*sqrt(1-ep^2))"
  Dot Product5/1 -> Display3/1, P1/1  "-2*(exp(-ep*wn*Ta))*cos(wn*Ta*sqrt(1-ep^2))"
  " "/1 -> Dot Product3/1
  [A] -> Dot Product7/1  "wn"
  Divide/1 -> Dot Product2/1, [A]  "wn"
  Math Function/1 -> Dot Product1/2  "e^(-ep*wn*Ta)"

== system rst_auto_reg_complete_4a_2018b/Auto-Ajuste/RST Degrau/Matrix M ==
  In1 : Inport
  " 1" : Constant  Value=0
  2 : Constant
  Demux : Demux  Outputs=8
  Display1 : Display
  Matrix Concatenate{1..8} (8 alike) : Concatenate  NumInputs=8  Mode=Multidimensional array  ConcatenateDimension=2
  Matrix Concatenate{9..15} (7 alike) : Concatenate  Mode=Multidimensional array
  M : Outport
  wires:
  Matrix Concatenate12/1 -> Matrix Concatenate14/1
  Matrix Concatenate13/1 -> Matrix Concatenate14/2
  Matrix Concatenate6/1 -> Matrix Concatenate12/1
  2/1 -> Matrix Concatenate3/4, Matrix Concatenate2/3, Matrix Concatenate1/2, Matrix Concatenate6/1  "1"
  In1/1 -> Demux/1
  " 1"/1 -> Matrix Concatenate8/7, Matrix Concatenate8/6, Matrix Concatenate8/5, Matrix Concatenate8/3, Matrix Concatenate8/2, Matrix Concatenate8/1, Matrix Concatenate7/6, Matrix Concatenate7/5, Matrix Concatenate7/2, Matrix Concatenate7/1, Matrix Concatenate5/5, Matrix Concatenate5/1, Matrix Concatenate3/8, Matrix Concatenate2/8, Matrix Concatenate2/7, Matrix Concatenate2/4, Matrix Concatenate1/8, Matrix Concatenate1/7, Matrix Concatenate1/6, Matrix Concatenate1/4, Matrix Concatenate1/3, Matrix Concatenate6/8, Matrix Concatenate6/7, Matrix Concatenate6/6, Matrix Concatenate6/5, Matrix Concatenate6/4, Matrix Concatenate6/3, Matrix Concatenate6/2  "0"
  Demux/1 -> Matrix Concatenate4/4, Matrix Concatenate3/3, Matrix Concatenate2/2, Matrix Concatenate1/1  "a1"
  Demux/2 -> Matrix Concatenate5/4, Matrix Concatenate4/3, Matrix Concatenate3/2, Matrix Concatenate2/1  "a2"
  Demux/3 -> Matrix Concatenate7/4, Matrix Concatenate5/3, Matrix Concatenate4/2, Matrix Concatenate3/1  "a3"
  Demux/4 -> Matrix Concatenate8/4, Matrix Concatenate7/3, Matrix Concatenate5/2, Matrix Concatenate4/1  "a4"
  Demux/5 -> Matrix Concatenate4/8, Matrix Concatenate3/7, Matrix Concatenate2/6, Matrix Concatenate1/5  "b1"
  Demux/6 -> Matrix Concatenate5/8, Matrix Concatenate4/7, Matrix Concatenate3/6, Matrix Concatenate2/5  "b2"
  Demux/7 -> Matrix Concatenate7/8, Matrix Concatenate5/7, Matrix Concatenate4/6, Matrix Concatenate3/5  "b3"
  Demux/8 -> Matrix Concatenate8/8, Matrix Concatenate7/7, Matrix Concatenate5/6, Matrix Concatenate4/5  "b4"
  Matrix Concatenate1/1 -> Matrix Concatenate12/2
  Matrix Concatenate2/1 -> Matrix Concatenate13/1
  Matrix Concatenate3/1 -> Matrix Concatenate13/2
  Matrix Concatenate4/1 -> Matrix Concatenate9/1
  Matrix Concatenate5/1 -> Matrix Concatenate9/2
  Matrix Concatenate7/1 -> Matrix Concatenate10/1
  Matrix Concatenate8/1 -> Matrix Concatenate10/2
  Matrix Concatenate10/1 -> Matrix Concatenate11/2
  Matrix Concatenate9/1 -> Matrix Concatenate11/1
  Matrix Concatenate11/1 -> Matrix Concatenate15/2
  Matrix Concatenate14/1 -> Matrix Concatenate15/1
  Matrix Concatenate15/1 -> M/1, Display1/1

== system rst_auto_reg_complete_4a_2018b/Auto-Ajuste/RST Degrau/Matrix Q ==
  P1 : Inport
  P2 : Inport  Port=2
  Constant : Constant
  Constant1 : Constant  Value=0
  Display1 : Display
  Matrix Concatenate{1..7} (7 alike) : Concatenate  Mode=Multidimensional array
  Q1 : Outport
  wires:
  Constant1/1 -> Matrix Concatenate5/2, Matrix Concatenate5/1, Matrix Concatenate4/2, Matrix Concatenate4/1, Matrix Concatenate3/2
  Constant/1 -> Matrix Concatenate1/1
  P1/1 -> Matrix Concatenate1/2
  P2/1 -> Matrix Concatenate3/1
  Matrix Concatenate3/1 -> Matrix Concatenate2/2
  Matrix Concatenate1/1 -> Matrix Concatenate2/1
  Matrix Concatenate4/1 -> Matrix Concatenate6/1
  Matrix Concatenate5/1 -> Matrix Concatenate6/2
  Matrix Concatenate6/1 -> Matrix Concatenate7/2
  Matrix Concatenate2/1 -> Matrix Concatenate7/1
  Matrix Concatenate7/1 -> Q1/1, Display1/1

== system rst_auto_reg_complete_4a_2018b/Auto-Ajuste/RST Degrau/Subsystem ==
  Theta : Inport
  0 : Constant  Value=0
  Demux : Demux  Outputs=8
  Display1 : Display
  Display3 : Display
  Matrix Concatenate{1,9,16..21} (8 alike) : Concatenate  NumInputs=8  Mode=Multidimensional array  ConcatenateDimension=2
  Matrix Concatenate{3,7..8,10..11,15,22} (7 alike) : Concatenate  Mode=Multidimensional array
  Mux : Mux
  X1(1) : Constant
  X1(2) : Constant  Value=-1
  M2 : Outport
  wires:
  Matrix Concatenate1/1 -> Matrix Concatenate3/2
  Matrix Concatenate20/1 -> Matrix Concatenate10/1
  Matrix Concatenate21/1 -> Matrix Concatenate10/2
  Matrix Concatenate10/1 -> Matrix Concatenate11/2
  Matrix Concatenate11/1 -> Matrix Concatenate15/2
  Matrix Concatenate22/1 -> Matrix Concatenate11/1
  Matrix Concatenate18/1 -> Matrix Concatenate22/2
  Matrix Concatenate9/1 -> Matrix Concatenate7/1
  Matrix Concatenate17/1 -> Matrix Concatenate22/1
  Matrix Concatenate8/1 -> Matrix Concatenate15/1
  Matrix Concatenate16/1 -> Matrix Concatenate7/2
  Theta/1 -> Demux/1
  Matrix Concatenate3/1 -> Matrix Concatenate8/1
  Matrix Concatenate7/1 -> Matrix Concatenate8/2
  Matrix Concatenate19/1 -> Matrix Concatenate3/1
  X1(1)/1 -> Matrix Concatenate16/4, Matrix Concatenate9/3, Matrix Concatenate1/2, Matrix Concatenate19/1  "X1(1)"
  Demux/1 -> Mux/1  "a1"
  Demux/2 -> Mux/2  "a2"
  Demux/3 -> Mux/3  "a3"
  Demux/4 -> Mux/4  "a4"
  Mux/1 -> Display3/1
  0/1 -> Matrix Concatenate19/5, Matrix Concatenate1/6, Matrix Concatenate9/7, Matrix Concatenate16/8, Matrix Concatenate20/4, Matrix Concatenate21/7, Matrix Concatenate21/6, Matrix Concatenate21/5, Matrix Concatenate21/4, Matrix Concatenate21/3, Matrix Concatenate21/2, Matrix Concatenate21/1, Matrix Concatenate20/6, Matrix Concatenate20/5, Matrix Concatenate20/3, Matrix Concatenate20/2, Matrix Concatenate20/1, Matrix Concatenate18/5, Matrix Concatenate18/4, Matrix Concatenate18/3, Matrix Concatenate18/2, Matrix Concatenate18/1, Matrix Concatenate17/3, Matrix Concatenate17/2, Matrix Concatenate17/1, Matrix Concatenate16/2, Matrix Concatenate16/1, Matrix Concatenate9/8, Matrix Concatenate9/4, Matrix Concatenate9/1, Matrix Concatenate1/8, Matrix Concatenate1/7, Matrix Concatenate1/4, Matrix Concatenate1/3, Matrix Concatenate19/8, Matrix Concatenate19/7, Matrix Concatenate19/6, Matrix Concatenate19/4, Matrix Concatenate19/3, Matrix Concatenate19/2  "0"
  Matrix Concatenate15/1 -> M2/1, Display1/1
  X1(2)/1 -> Matrix Concatenate17/4, Matrix Concatenate16/3, Matrix Concatenate9/2, Matrix Concatenate1/1  "X1(2)"
  Demux/5 -> Matrix Concatenate17/8, Matrix Concatenate16/7, Matrix Concatenate9/6, Matrix Concatenate1/5  "b2"
  Demux/6 -> Matrix Concatenate18/8, Matrix Concatenate17/7, Matrix Concatenate16/6, Matrix Concatenate9/5  "b3"
  Demux/7 -> Matrix Concatenate20/8, Matrix Concatenate18/7, Matrix Concatenate17/6, Matrix Concatenate16/5  "b4"
  Demux/8 -> Matrix Concatenate21/8, Matrix Concatenate20/7, Matrix Concatenate18/6, Matrix Concatenate17/5  "b5"

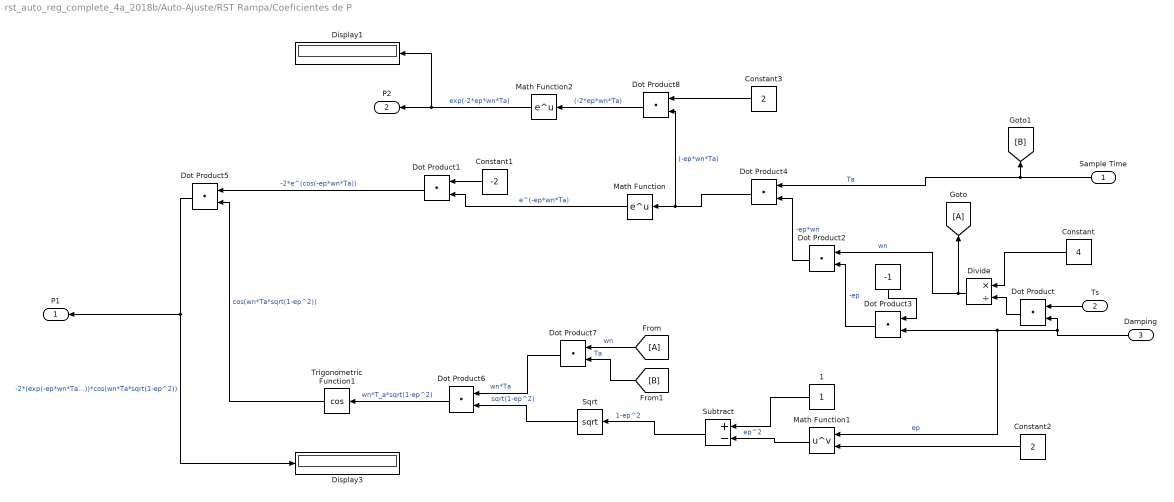
== system rst_auto_reg_complete_4a_2018b/Auto-Ajuste/RST Rampa/Coeficientes de P ==
  Sample Time : Inport
  Ts : Inport  Port=2
  Damping : Inport  Port=3
  " " : Constant  Value=-1
  1 : Constant
  Constant : Constant  Value=4
  Constant1 : Constant  Value=-2
  Constant2 : Constant  Value=2
  Constant3 : Constant  Value=2
  Display1 : Display
  Display3 : Display
  Divide : Product  Inputs=*/
  Dot Product{,1..8} (9 alike) : DotProduct  InputSameDT=on  OutDataTypeStr=Inherit: Inherit via internal rule
  Math Function : Math  SaturateOnIntegerOverflow=on
  Math Function1 : Math  Operator=pow  SaturateOnIntegerOverflow=on
  Math Function2 : Math  SaturateOnIntegerOverflow=on
  Sqrt : Sqrt  SaturateOnIntegerOverflow=on
  Subtract : Sum  Inputs=+-
  Trigonometric Function1 : Trigonometry  Operator=cos
  P1 : Outport
  P2 : Outport  Port=2
  wires:
  Math Function/1 -> Dot Product1/2  "e^(-ep*wn*Ta)"
  Divide/1 -> [A], Dot Product2/1  "wn"
  [A] -> Dot Product7/1  "wn"
  " "/1 -> Dot Product3/1
  Dot Product5/1 -> P1/1, Display3/1  "-2*(exp(-ep*wn*Ta))*cos(wn*Ta*sqrt(1-ep^2))"
  Trigonometric Function1/1 -> Dot Product5/2  "cos(wn*Ta*sqrt(1-ep^2))"
  Ts/1 -> Dot Product/1
  Dot Product/1 -> Divide/2
  Dot Product3/1 -> Dot Product2/2  "-ep"
  Damping/1 -> Math Function1/1, Dot Product3/2, Dot Product/2  "ep"
  Constant/1 -> Divide/1
  Dot Product7/1 -> Dot Product6/1  "wn*Ta"
  Sample Time/1 -> Dot Product4/1, [B]  "Ta"
  Math Function1/1 -> Subtract/2  "ep^2"
  Dot Product1/1 -> Dot Product5/1  "-2*e^(cos(-ep*wn*Ta))"
  Constant2/1 -> Math Function1/2
  1/1 -> Subtract/1
  Constant1/1 -> Dot Product1/1
  Dot Product2/1 -> Dot Product4/2  "-ep*wn"
  [B] -> Dot Product7/2  "Ta"
  Dot Product6/1 -> Trigonometric Function1/1  "wn*T_a*sqrt(1-ep^2)"
  Dot Product4/1 -> Dot Product8/2, Math Function/1  "(-ep*wn*Ta)"
  Sqrt/1 -> Dot Product6/2  "sqrt(1-ep^2)"
  Subtract/1 -> Sqrt/1  "1-ep^2"
  Constant3/1 -> Dot Product8/1
  Dot Product8/1 -> Math Function2/1  "(-2*ep*wn*Ta)"
  Math Function2/1 -> Display1/1, P2/1  "exp(-2*ep*wn*Ta)"

== system rst_auto_reg_complete_4a_2018b/Auto-Ajuste/RST Rampa/Matrix M1 ==
  In1 : Inport
  " 1" : Constant  Value=0
  2 : Constant
  Demux : Demux  Outputs=8
  Display1 : Display
  Matrix Concatenate{1..8} (8 alike) : Concatenate  NumInputs=8  Mode=Multidimensional array  ConcatenateDimension=2
  Matrix Concatenate{9..15} (7 alike) : Concatenate  Mode=Multidimensional array
  M : Outport
  wires:
  Matrix Concatenate12/1 -> Matrix Concatenate14/1
  Matrix Concatenate13/1 -> Matrix Concatenate14/2
  Matrix Concatenate6/1 -> Matrix Concatenate12/1
  2/1 -> Matrix Concatenate3/4, Matrix Concatenate2/3, Matrix Concatenate1/2, Matrix Concatenate6/1  "1"
  In1/1 -> Demux/1
  " 1"/1 -> Matrix Concatenate8/7, Matrix Concatenate8/6, Matrix Concatenate8/5, Matrix Concatenate8/3, Matrix Concatenate8/2, Matrix Concatenate8/1, Matrix Concatenate7/6, Matrix Concatenate7/5, Matrix Concatenate7/2, Matrix Concatenate7/1, Matrix Concatenate5/5, Matrix Concatenate5/1, Matrix Concatenate3/8, Matrix Concatenate2/8, Matrix Concatenate2/7, Matrix Concatenate2/4, Matrix Concatenate1/8, Matrix Concatenate1/7, Matrix Concatenate1/6, Matrix Concatenate1/4, Matrix Concatenate1/3, Matrix Concatenate6/8, Matrix Concatenate6/7, Matrix Concatenate6/6, Matrix Concatenate6/5, Matrix Concatenate6/4, Matrix Concatenate6/3, Matrix Concatenate6/2  "0"
  Demux/1 -> Matrix Concatenate4/4, Matrix Concatenate3/3, Matrix Concatenate2/2, Matrix Concatenate1/1  "a1"
  Demux/2 -> Matrix Concatenate5/4, Matrix Concatenate4/3, Matrix Concatenate3/2, Matrix Concatenate2/1  "a2"
  Demux/3 -> Matrix Concatenate7/4, Matrix Concatenate5/3, Matrix Concatenate4/2, Matrix Concatenate3/1  "a3"
  Demux/4 -> Matrix Concatenate8/4, Matrix Concatenate7/3, Matrix Concatenate5/2, Matrix Concatenate4/1  "a4"
  Demux/5 -> Matrix Concatenate4/8, Matrix Concatenate3/7, Matrix Concatenate2/6, Matrix Concatenate1/5  "b1"
  Demux/6 -> Matrix Concatenate5/8, Matrix Concatenate4/7, Matrix Concatenate3/6, Matrix Concatenate2/5  "b2"
  Demux/7 -> Matrix Concatenate7/8, Matrix Concatenate5/7, Matrix Concatenate4/6, Matrix Concatenate3/5  "b3"
  Demux/8 -> Matrix Concatenate8/8, Matrix Concatenate7/7, Matrix Concatenate5/6, Matrix Concatenate4/5  "b4"
  Matrix Concatenate1/1 -> Matrix Concatenate12/2
  Matrix Concatenate2/1 -> Matrix Concatenate13/1
  Matrix Concatenate3/1 -> Matrix Concatenate13/2
  Matrix Concatenate4/1 -> Matrix Concatenate9/1
  Matrix Concatenate5/1 -> Matrix Concatenate9/2
  Matrix Concatenate7/1 -> Matrix Concatenate10/1
  Matrix Concatenate8/1 -> Matrix Concatenate10/2
  Matrix Concatenate10/1 -> Matrix Concatenate11/2
  Matrix Concatenate9/1 -> Matrix Concatenate11/1
  Matrix Concatenate11/1 -> Matrix Concatenate15/2
  Matrix Concatenate14/1 -> Matrix Concatenate15/1
  Matrix Concatenate15/1 -> M/1, Display1/1

== system rst_auto_reg_complete_4a_2018b/Auto-Ajuste/RST Rampa/Matrix Q1 ==
  P1 : Inport
  P2 : Inport  Port=2
  Constant : Constant
  Constant1 : Constant  Value=0
  Display1 : Display
  Matrix Concatenate{1..7} (7 alike) : Concatenate  Mode=Multidimensional array
  Q1 : Outport
  wires:
  Constant1/1 -> Matrix Concatenate5/2, Matrix Concatenate5/1, Matrix Concatenate4/2, Matrix Concatenate4/1, Matrix Concatenate3/2
  Constant/1 -> Matrix Concatenate1/1
  P1/1 -> Matrix Concatenate1/2
  P2/1 -> Matrix Concatenate3/1
  Matrix Concatenate3/1 -> Matrix Concatenate2/2
  Matrix Concatenate1/1 -> Matrix Concatenate2/1
  Matrix Concatenate4/1 -> Matrix Concatenate6/1
  Matrix Concatenate5/1 -> Matrix Concatenate6/2
  Matrix Concatenate6/1 -> Matrix Concatenate7/2
  Matrix Concatenate2/1 -> Matrix Concatenate7/1
  Matrix Concatenate7/1 -> Q1/1, Display1/1

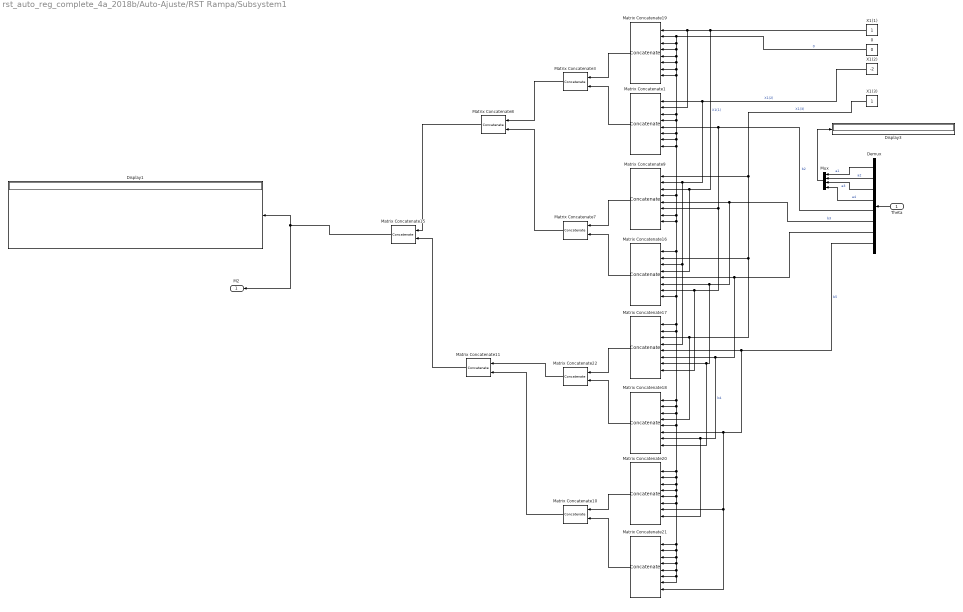
== system rst_auto_reg_complete_4a_2018b/Auto-Ajuste/RST Rampa/Subsystem1 ==
  Theta : Inport
  0 : Constant  Value=0
  Demux : Demux  Outputs=8
  Display1 : Display
  Display3 : Display
  Matrix Concatenate{1,9,16..21} (8 alike) : Concatenate  NumInputs=8  Mode=Multidimensional array  ConcatenateDimension=2
  Matrix Concatenate{3,7..8,10..11,15,22} (7 alike) : Concatenate  Mode=Multidimensional array
  Mux : Mux
  X1(1) : Constant
  X1(2) : Constant  Value=-2
  X1(3) : Constant
  M2 : Outport
  wires:
  Matrix Concatenate1/1 -> Matrix Concatenate3/2
  Matrix Concatenate20/1 -> Matrix Concatenate10/1
  Matrix Concatenate21/1 -> Matrix Concatenate10/2
  Matrix Concatenate10/1 -> Matrix Concatenate11/2
  Matrix Concatenate11/1 -> Matrix Concatenate15/2
  Matrix Concatenate22/1 -> Matrix Concatenate11/1
  Matrix Concatenate18/1 -> Matrix Concatenate22/2
  Matrix Concatenate9/1 -> Matrix Concatenate7/1
  Matrix Concatenate17/1 -> Matrix Concatenate22/1
  Matrix Concatenate8/1 -> Matrix Concatenate15/1
  Matrix Concatenate16/1 -> Matrix Concatenate7/2
  Theta/1 -> Demux/1
  Matrix Concatenate3/1 -> Matrix Concatenate8/1
  Matrix Concatenate7/1 -> Matrix Concatenate8/2
  Matrix Concatenate19/1 -> Matrix Concatenate3/1
  X1(1)/1 -> Matrix Concatenate16/4, Matrix Concatenate9/3, Matrix Concatenate1/2, Matrix Concatenate19/1  "X1(1)"
  Demux/1 -> Mux/1  "a1"
  Demux/2 -> Mux/2  "a2"
  Demux/3 -> Mux/3  "a3"
  Demux/4 -> Mux/4  "a4"
  Mux/1 -> Display3/1
  0/1 -> Matrix Concatenate19/5, Matrix Concatenate1/6, Matrix Concatenate9/7, Matrix Concatenate16/8, Matrix Concatenate20/4, Matrix Concatenate21/7, Matrix Concatenate21/6, Matrix Concatenate21/5, Matrix Concatenate21/4, Matrix Concatenate21/3, Matrix Concatenate21/2, Matrix Concatenate21/1, Matrix Concatenate20/6, Matrix Concatenate20/5, Matrix Concatenate20/3, Matrix Concatenate20/2, Matrix Concatenate20/1, Matrix Concatenate18/5, Matrix Concatenate18/3, Matrix Concatenate18/2, Matrix Concatenate18/1, Matrix Concatenate17/2, Matrix Concatenate17/1, Matrix Concatenate16/1, Matrix Concatenate9/8, Matrix Concatenate9/4, Matrix Concatenate1/8, Matrix Concatenate1/7, Matrix Concatenate1/4, Matrix Concatenate1/3, Matrix Concatenate19/8, Matrix Concatenate19/7, Matrix Concatenate19/6, Matrix Concatenate19/4, Matrix Concatenate19/3, Matrix Concatenate19/2  "0"
  Matrix Concatenate15/1 -> M2/1, Display1/1
  X1(2)/1 -> Matrix Concatenate17/4, Matrix Concatenate16/3, Matrix Concatenate9/2, Matrix Concatenate1/1  "X1(2)"
  Demux/5 -> Matrix Concatenate17/8, Matrix Concatenate16/7, Matrix Concatenate9/6, Matrix Concatenate1/5  "b2"
  Demux/6 -> Matrix Concatenate18/8, Matrix Concatenate17/7, Matrix Concatenate16/6, Matrix Concatenate9/5  "b3"
  Demux/7 -> Matrix Concatenate20/8, Matrix Concatenate18/7, Matrix Concatenate17/6, Matrix Concatenate16/5  "b4"
  Demux/8 -> Matrix Concatenate21/8, Matrix Concatenate20/7, Matrix Concatenate18/6, Matrix Concatenate17/5  "b5"
  X1(3)/1 -> Matrix Concatenate18/4, Matrix Concatenate17/3, Matrix Concatenate16/2, Matrix Concatenate9/1  "X1(3)"

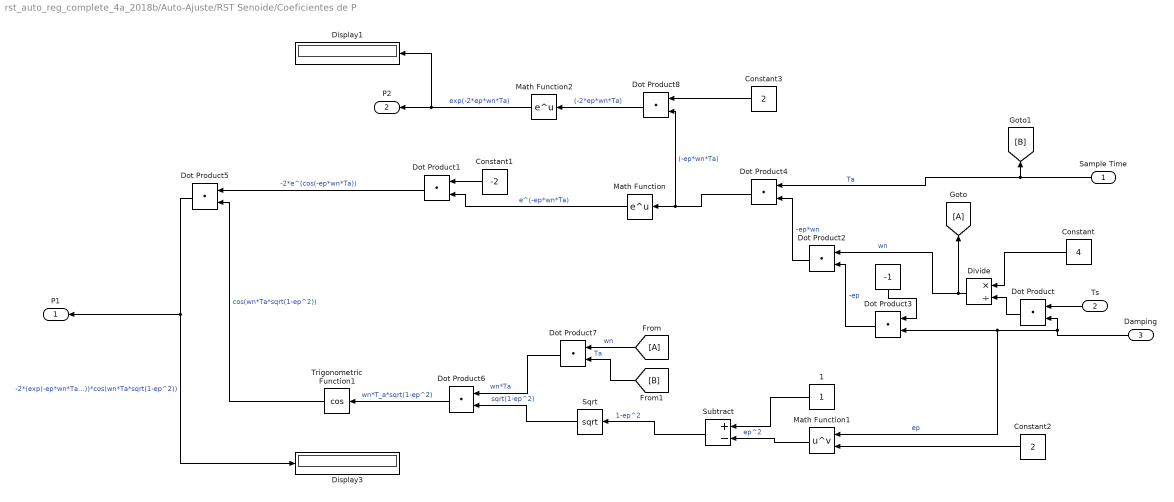
== system rst_auto_reg_complete_4a_2018b/Auto-Ajuste/RST Senoide/Coeficientes de P ==
  Sample Time : Inport
  Ts : Inport  Port=2
  Damping : Inport  Port=3
  " " : Constant  Value=-1
  1 : Constant
  Constant : Constant  Value=4
  Constant1 : Constant  Value=-2
  Constant2 : Constant  Value=2
  Constant3 : Constant  Value=2
  Display1 : Display
  Display3 : Display
  Divide : Product  Inputs=*/
  Dot Product{,1..8} (9 alike) : DotProduct  InputSameDT=on  OutDataTypeStr=Inherit: Inherit via internal rule
  Math Function : Math  SaturateOnIntegerOverflow=on
  Math Function1 : Math  Operator=pow  SaturateOnIntegerOverflow=on
  Math Function2 : Math  SaturateOnIntegerOverflow=on
  Sqrt : Sqrt  SaturateOnIntegerOverflow=on
  Subtract : Sum  Inputs=+-
  Trigonometric Function1 : Trigonometry  Operator=cos
  P1 : Outport
  P2 : Outport  Port=2
  wires:
  Math Function/1 -> Dot Product1/2  "e^(-ep*wn*Ta)"
  Divide/1 -> [A], Dot Product2/1  "wn"
  [A] -> Dot Product7/1  "wn"
  " "/1 -> Dot Product3/1
  Dot Product5/1 -> P1/1, Display3/1  "-2*(exp(-ep*wn*Ta))*cos(wn*Ta*sqrt(1-ep^2))"
  Trigonometric Function1/1 -> Dot Product5/2  "cos(wn*Ta*sqrt(1-ep^2))"
  Ts/1 -> Dot Product/1
  Dot Product/1 -> Divide/2
  Dot Product3/1 -> Dot Product2/2  "-ep"
  Damping/1 -> Math Function1/1, Dot Product3/2, Dot Product/2  "ep"
  Constant/1 -> Divide/1
  Dot Product7/1 -> Dot Product6/1  "wn*Ta"
  Sample Time/1 -> Dot Product4/1, [B]  "Ta"
  Math Function1/1 -> Subtract/2  "ep^2"
  Dot Product1/1 -> Dot Product5/1  "-2*e^(cos(-ep*wn*Ta))"
  Constant2/1 -> Math Function1/2
  1/1 -> Subtract/1
  Constant1/1 -> Dot Product1/1
  Dot Product2/1 -> Dot Product4/2  "-ep*wn"
  [B] -> Dot Product7/2  "Ta"
  Dot Product6/1 -> Trigonometric Function1/1  "wn*T_a*sqrt(1-ep^2)"
  Dot Product4/1 -> Dot Product8/2, Math Function/1  "(-ep*wn*Ta)"
  Sqrt/1 -> Dot Product6/2  "sqrt(1-ep^2)"
  Subtract/1 -> Sqrt/1  "1-ep^2"
  Constant3/1 -> Dot Product8/1
  Dot Product8/1 -> Math Function2/1  "(-2*ep*wn*Ta)"
  Math Function2/1 -> Display1/1, P2/1  "exp(-2*ep*wn*Ta)"

== system rst_auto_reg_complete_4a_2018b/Auto-Ajuste/RST Senoide/Matrix M1 ==
  In1 : Inport
  " 1" : Constant  Value=0
  2 : Constant
  Demux : Demux  Outputs=8
  Display1 : Display
  Matrix Concatenate{1..8} (8 alike) : Concatenate  NumInputs=8  Mode=Multidimensional array  ConcatenateDimension=2
  Matrix Concatenate{9..15} (7 alike) : Concatenate  Mode=Multidimensional array
  M : Outport
  wires:
  Matrix Concatenate12/1 -> Matrix Concatenate14/1
  Matrix Concatenate13/1 -> Matrix Concatenate14/2
  Matrix Concatenate6/1 -> Matrix Concatenate12/1
  2/1 -> Matrix Concatenate3/4, Matrix Concatenate2/3, Matrix Concatenate1/2, Matrix Concatenate6/1  "1"
  In1/1 -> Demux/1
  " 1"/1 -> Matrix Concatenate8/7, Matrix Concatenate8/6, Matrix Concatenate8/5, Matrix Concatenate8/3, Matrix Concatenate8/2, Matrix Concatenate8/1, Matrix Concatenate7/6, Matrix Concatenate7/5, Matrix Concatenate7/2, Matrix Concatenate7/1, Matrix Concatenate5/5, Matrix Concatenate5/1, Matrix Concatenate3/8, Matrix Concatenate2/8, Matrix Concatenate2/7, Matrix Concatenate2/4, Matrix Concatenate1/8, Matrix Concatenate1/7, Matrix Concatenate1/6, Matrix Concatenate1/4, Matrix Concatenate1/3, Matrix Concatenate6/8, Matrix Concatenate6/7, Matrix Concatenate6/6, Matrix Concatenate6/5, Matrix Concatenate6/4, Matrix Concatenate6/3, Matrix Concatenate6/2  "0"
  Demux/1 -> Matrix Concatenate4/4, Matrix Concatenate3/3, Matrix Concatenate2/2, Matrix Concatenate1/1  "a1"
  Demux/2 -> Matrix Concatenate5/4, Matrix Concatenate4/3, Matrix Concatenate3/2, Matrix Concatenate2/1  "a2"
  Demux/3 -> Matrix Concatenate7/4, Matrix Concatenate5/3, Matrix Concatenate4/2, Matrix Concatenate3/1  "a3"
  Demux/4 -> Matrix Concatenate8/4, Matrix Concatenate7/3, Matrix Concatenate5/2, Matrix Concatenate4/1  "a4"
  Demux/5 -> Matrix Concatenate4/8, Matrix Concatenate3/7, Matrix Concatenate2/6, Matrix Concatenate1/5  "b1"
  Demux/6 -> Matrix Concatenate5/8, Matrix Concatenate4/7, Matrix Concatenate3/6, Matrix Concatenate2/5  "b2"
  Demux/7 -> Matrix Concatenate7/8, Matrix Concatenate5/7, Matrix Concatenate4/6, Matrix Concatenate3/5  "b3"
  Demux/8 -> Matrix Concatenate8/8, Matrix Concatenate7/7, Matrix Concatenate5/6, Matrix Concatenate4/5  "b4"
  Matrix Concatenate1/1 -> Matrix Concatenate12/2
  Matrix Concatenate2/1 -> Matrix Concatenate13/1
  Matrix Concatenate3/1 -> Matrix Concatenate13/2
  Matrix Concatenate4/1 -> Matrix Concatenate9/1
  Matrix Concatenate5/1 -> Matrix Concatenate9/2
  Matrix Concatenate7/1 -> Matrix Concatenate10/1
  Matrix Concatenate8/1 -> Matrix Concatenate10/2
  Matrix Concatenate10/1 -> Matrix Concatenate11/2
  Matrix Concatenate9/1 -> Matrix Concatenate11/1
  Matrix Concatenate11/1 -> Matrix Concatenate15/2
  Matrix Concatenate14/1 -> Matrix Concatenate15/1
  Matrix Concatenate15/1 -> M/1, Display1/1

== system rst_auto_reg_complete_4a_2018b/Auto-Ajuste/RST Senoide/Matrix Q ==
  P1 : Inport
  P2 : Inport  Port=2
  Constant : Constant
  Constant1 : Constant  Value=0
  Display1 : Display
  Matrix Concatenate{1..7} (7 alike) : Concatenate  Mode=Multidimensional array
  Q1 : Outport
  wires:
  Constant1/1 -> Matrix Concatenate5/2, Matrix Concatenate5/1, Matrix Concatenate4/2, Matrix Concatenate4/1, Matrix Concatenate3/2
  Constant/1 -> Matrix Concatenate1/1
  P1/1 -> Matrix Concatenate1/2
  P2/1 -> Matrix Concatenate3/1
  Matrix Concatenate3/1 -> Matrix Concatenate2/2
  Matrix Concatenate1/1 -> Matrix Concatenate2/1
  Matrix Concatenate4/1 -> Matrix Concatenate6/1
  Matrix Concatenate5/1 -> Matrix Concatenate6/2
  Matrix Concatenate6/1 -> Matrix Concatenate7/2
  Matrix Concatenate2/1 -> Matrix Concatenate7/1
  Matrix Concatenate7/1 -> Q1/1, Display1/1
